simulink model "Projectslxfinal"  (R2021b)
settings: Solver=VariableStepAuto  StartTime=0.0  StopTime=0.01  RelTol=1e-3
undefined symbols (not defined in the file): A_d, B_d, C_d, k, L
libraries: simulink x3, slpidlib x3
settings Model: Creator=hp  LastModifiedBy=mahya
settings DataIOCC: ExternalInput=T1, T2, T3, Gdz1.Numerator{1,1}, Gdz1.Denominator{1,1}, Gdz2.Numerator{1,1}, Gdz2.Denominator{1,1}, Gdz3.Numerator{1,1}, Gdz3.Denominator{1,1}

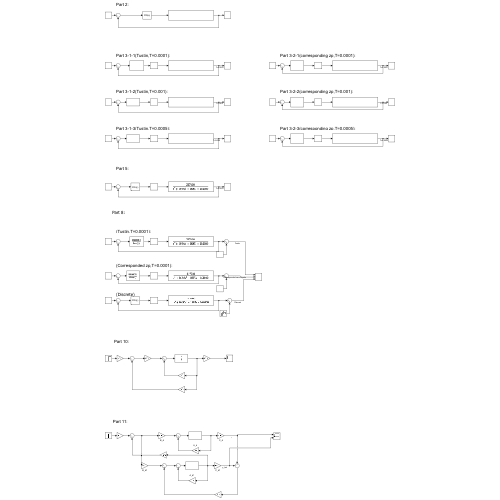
[thumbnail: Simulink's stored preview of the top-level diagram]
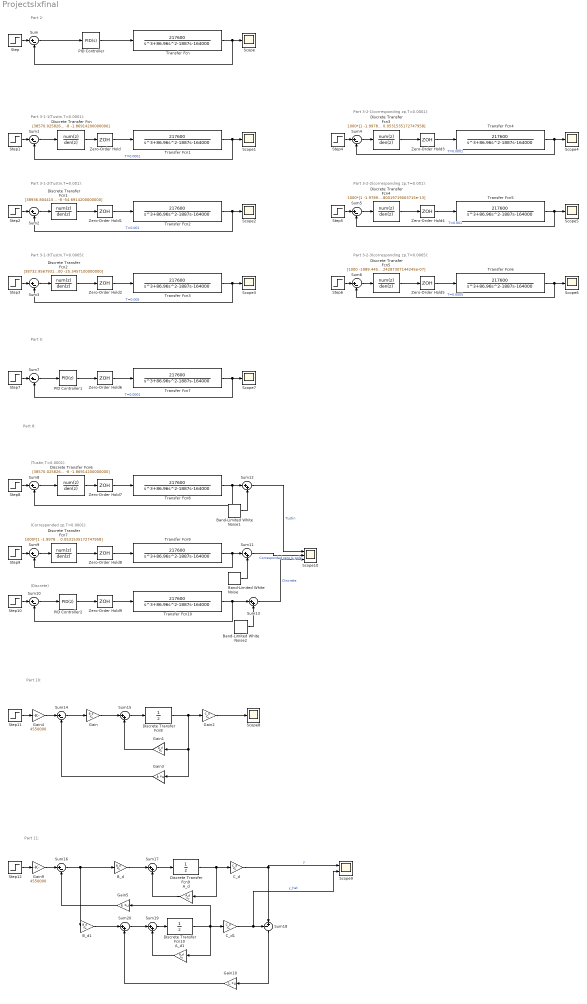
== system Projectslxfinal ==
  note: (Discrete)
  note: Part 8:
  note: Part 5:
  note: Part 2:
  note: Part 3-1-2(Tustin,T=0.001):
  note: Part 3-1-3(Tustin,T=0.0005):
  note: Part 3-2-1(corresponding zp,T=0.0001):
  note: Part 3-1-1(Tustin,T=0.0001):
  note: Part 3-2-2(corresponding zp,T=0.001):
  note: Part 3-2-3(corresponding zp,T=0.0005):
  note: (Corresponded zp,T=0.0001):
  note: (Tustin,T=0.0001):
  note: Part 10:
  note: Part 11:
  A_d : Gain  Gain=A_d  Multiplication=Matrix(K*u)
  A_d1 : Gain  Gain=A_d  Multiplication=Matrix(K*u)
  B_d : Gain  Gain=B_d  Multiplication=Matrix(K*u)
  B_d1 : Gain  Gain=B_d  Multiplication=Matrix(K*u)
  Band-Limited White Noise : simulink/Sources/Band-Limited White Noise  Cov=[0.00001]  Ts=0.1  seed=[23341]
  Band-Limited White Noise1 : simulink/Sources/Band-Limited White Noise  Cov=[0.00001]  Ts=0.1  seed=[23341]
  Band-Limited White Noise2 : simulink/Sources/Band-Limited White Noise  Cov=[0.00001]  Ts=0.1  seed=[23341]
  C_d : Gain  Gain=C_d  Multiplication=Matrix(K*u)
  C_d1 : Gain  Gain=C_d  Multiplication=Matrix(K*u)
  Discrete Transfer Fcn : DiscreteTransferFcn  Numerator=[38570.0258267180 -77058.6188660459 38488.6093872360]  Denominator=[9.86914200000000 -8 -1.86914200000000]  SampleTime=0.0001
  Discrete Transfer Fcn1 : DiscreteTransferFcn  Numerator=[38936.8044151132 -77057.8096445937 38122.6400202932]  Denominator=[62.6914200000000 -8 -54.6914200000000]  SampleTime=0.001
  Discrete Transfer Fcn10 : DiscreteTransferFcn  Denominator=[1 0]
  Discrete Transfer Fcn2 : DiscreteTransferFcn  Numerator=[38732.9567931308 -77058.4226911484 38325.8745957208]  Denominator=[33.3457100000000 -8.00000000000000 -25.3457100000000]  SampleTime=0.0005
  Discrete Transfer Fcn3 : DiscreteTransferFcn  Numerator=1000*[1 -1.99788732081826 0.997889127214699]  Denominator=[1 -1.05315351727480 0.0531535172747958]  SampleTime=0.0001
  Discrete Transfer Fcn4 : DiscreteTransferFcn  Numerator=1000*[1 -1.97891172719588 0.979090657910839]  Denominator=[1 -1.00000000000018 1.80019719003715e-13]  SampleTime=0.001
  Discrete Transfer Fcn5 : DiscreteTransferFcn  Numerator=[1000 -1989.44513045919 989.490099955951]  Denominator=[1 -1.00000042428731 4.24287307144245e-07]  SampleTime=0.0005
  Discrete Transfer Fcn6 : DiscreteTransferFcn  Numerator=[38570.0258267180 -77058.6188660459 38488.6093872360]  Denominator=[9.86914200000000 -8 -1.86914200000000]  SampleTime=0.0001
  Discrete Transfer Fcn7 : DiscreteTransferFcn  Numerator=1000*[1 -1.99788732081826 0.997889127214699]  Denominator=[1 -1.05315351727480 0.0531535172747958]  SampleTime=0.0001
  Discrete Transfer Fcn8 : DiscreteTransferFcn  Denominator=[1 0]
  Discrete Transfer Fcn9 : DiscreteTransferFcn  Denominator=[1 0]
  Gain : Gain  Gain=B_d  Multiplication=Matrix(K*u)
  Gain1 : Gain  Gain=A_d  Multiplication=Matrix(K*u)
  Gain10 : Gain  Gain=L  Multiplication=Matrix(K*u)
  Gain2 : Gain  Gain=C_d  Multiplication=Matrix(K*u)
  Gain3 : Gain  Gain=k  Multiplication=Matrix(K*u)
  Gain4 : Gain  Gain=4550000
  Gain5 : Gain  Gain=k  Multiplication=Matrix(K*u)
  Gain9 : Gain  Gain=4550000
  PID Controller : slpidlib/PID Controller  Controller=PID  Form=Parallel  TimeDomain=Continuous-time  UseExternalTs=off  SampleTime=-1  IntegratorMethod=Forward Euler  FilterMethod=Forward Euler  ControllerParametersSource=internal  P=6.93550294613259  I=13.9271022614454  D=0.32804013853127  UseFilter=on  N=29345.7140521187  TunerSelectOption=Transfer Function Based (PID Tuner App)  ZeroCross=off  InitialConditionSource=internal  InitialConditionForIntegrator=0  InitialConditionForFilter=0  DifferentiatorICPrevScaledInput=0  ExternalReset=none  TrackingMode=off  Kt=1  LimitOutput=off  SatLimitsSource=internal  UpperSaturationLimit=inf  LowerSaturationLimit=-inf  LinearizeAsGain=on  AntiWindupMode=none  Kb=1  POutMin=[]  POutMax=[]  IOutMin=[]  IOutMax=[]  DOutMin=[]  DOutMax=[]  NOutMin=[]  NOutMax=[]  SumOutMin=[]  SumOutMax=[]  SaturationOutMin=[]  SaturationOutMax=[]  PParamMin=[]  PParamMax=[]  IParamMin=[]  IParamMax=[]  DParamMin=[]  DParamMax=[]  NParamMin=[]  NParamMax=[]  KbParamMin=[]  KbParamMax=[]  KtParamMin=[]  KtParamMax=[]  KbOutMin=[]  KbOutMax=[]  KtOutMin=[]  KtOutMax=[]  IntegratorOutMin=[]  IntegratorOutMax=[]  FilterOutMin=[]  FilterOutMax=[]  SumI1OutMin=[]  SumI1OutMax=[]  SumI2OutMin=[]  SumI2OutMax=[]  SumI3OutMin=[]  SumI3OutMax=[]  SumI4OutMin=[]  SumI4OutMax=[]  SumDOutMin=[]  SumDOutMax=[]  DifferentiatorOutMin=[]  DifferentiatorOutMax=[]  FilterDiffOutCoefMin=[]  FilterDiffOutCoefMax=[]  ReciprocalOutMin=[]  ReciprocalOutMax=[]  SumDenOutMin=[]  SumDenOutMax=[]  SumNumOutMin=[]  SumNumOutMax=[]  DivideOutMin=[]  DivideOutMax=[]  UdiffTsProdOutMin=[]  UdiffTsProdOutMax=[]  NTsProdOutMin=[]  NTsProdOutMax=[]  UintegralTsProdOutMin=[]  UintegralTsProdOutMax=[]  UngainTsProdOutMin=[]  UngainTsProdOutMax=[]  IntegratorContinuousStateAttributes=''  IntegratorStateMustResolveToSignalObject=off  IntegratorRTWStateStorageClass=Auto  FilterContinuousStateAttributes=''  FilterStateMustResolveToSignalObject=off  FilterRTWStateStorageClass=Auto  ParallelPVariant=InternalParameters  IdealPVariant=Disabled  IVariant=InternalParameters  DVariant=InternalParameters  IntegratorVariant=Continuous  SatVariant=Disabled  AWVariant=Passthrough  PCopyVariant=Disabled  TRVariant=Disabled  FdbkBlocksVariant=Forward  IdealPFdbkVariant=Disabled  SatFdbkVariant=Disabled  DerivativeFilterVariant=ContFilter  NVariant=InternalParameters  NCopyVariant=Disabled  FilterICVariant=InternalICsFilter  IntegratorICVariant=InternalICs  ExternalResetVariant=Disabled  TRSumVariant=Passthrough  SumFdbkVariant=Disabled  SumVariant=Sum_PID  TsampFilterVariant=InternalTs  TsampNgainVariant=Passthrough  TsampIntegralVariant=Passthrough  ExternalSaturationOutDataTypeStr=Inherit: Same as second input
  PID Controller1 : slpidlib/PID Controller  Controller=PID  Form=Parallel  TimeDomain=Discrete-time  UseExternalTs=off  SampleTime=0.0001  IntegratorMethod=Forward Euler  FilterMethod=Forward Euler  ControllerParametersSource=internal  P=11.3216587748334  I=29.7415043652461  D=0.957335288291549  UseFilter=on  N=14403.0185628453  TunerSelectOption=Transfer Function Based (PID Tuner App)  InitialConditionSource=internal  InitialConditionForIntegrator=0  InitialConditionForFilter=0  DifferentiatorICPrevScaledInput=0  ExternalReset=none  TrackingMode=off  Kt=1  LimitOutput=off  SatLimitsSource=internal  UpperSaturationLimit=inf  LowerSaturationLimit=-inf  LinearizeAsGain=on  AntiWindupMode=none  Kb=1  POutMin=[]  POutMax=[]  IOutMin=[]  IOutMax=[]  DOutMin=[]  DOutMax=[]  NOutMin=[]  NOutMax=[]  SumOutMin=[]  SumOutMax=[]  SaturationOutMin=[]  SaturationOutMax=[]  PParamMin=[]  PParamMax=[]  IParamMin=[]  IParamMax=[]  DParamMin=[]  DParamMax=[]  NParamMin=[]  NParamMax=[]  KbParamMin=[]  KbParamMax=[]  KtParamMin=[]  KtParamMax=[]  KbOutMin=[]  KbOutMax=[]  KtOutMin=[]  KtOutMax=[]  IntegratorOutMin=[]  IntegratorOutMax=[]  FilterOutMin=[]  FilterOutMax=[]  SumI1OutMin=[]  SumI1OutMax=[]  SumI2OutMin=[]  SumI2OutMax=[]  SumI3OutMin=[]  SumI3OutMax=[]  SumI4OutMin=[]  SumI4OutMax=[]  SumDOutMin=[]  SumDOutMax=[]  DifferentiatorOutMin=[]  DifferentiatorOutMax=[]  FilterDiffOutCoefMin=[]  FilterDiffOutCoefMax=[]  ReciprocalOutMin=[]  ReciprocalOutMax=[]  SumDenOutMin=[]  SumDenOutMax=[]  SumNumOutMin=[]  SumNumOutMax=[]  DivideOutMin=[]  DivideOutMax=[]  UdiffTsProdOutMin=[]  UdiffTsProdOutMax=[]  NTsProdOutMin=[]  NTsProdOutMax=[]  UintegralTsProdOutMin=[]  UintegralTsProdOutMax=[]  UngainTsProdOutMin=[]  UngainTsProdOutMax=[]  IntegratorContinuousStateAttributes=''  IntegratorStateMustResolveToSignalObject=off  IntegratorRTWStateStorageClass=Auto  FilterContinuousStateAttributes=''  FilterStateMustResolveToSignalObject=off  FilterRTWStateStorageClass=Auto  ParallelPVariant=InternalParameters  IdealPVariant=Disabled  IVariant=InternalParameters  DVariant=InternalParameters  IntegratorVariant=Discrete  SatVariant=Disabled  AWVariant=Passthrough  PCopyVariant=Disabled  TRVariant=Disabled  FdbkBlocksVariant=Forward  IdealPFdbkVariant=Disabled  SatFdbkVariant=Disabled  DerivativeFilterVariant=ForwardEulerFilter  NVariant=InternalParameters  NCopyVariant=Disabled  FilterICVariant=InternalICsFilter  IntegratorICVariant=InternalICs  ExternalResetVariant=Disabled  TRSumVariant=Passthrough  SumFdbkVariant=Disabled  SumVariant=Sum_PID  TsampFilterVariant=InternalTs  TsampNgainVariant=Passthrough  TsampIntegralVariant=Passthrough  ExternalSaturationOutDataTypeStr=Inherit: Same as second input
  PID Controller2 : slpidlib/PID Controller  Controller=PID  Form=Parallel  TimeDomain=Discrete-time  UseExternalTs=off  SampleTime=0.0001  IntegratorMethod=Forward Euler  FilterMethod=Forward Euler  ControllerParametersSource=internal  P=11.3216587748334  I=29.7415043652461  D=0.957335288291549  UseFilter=on  N=14403.0185628453  TunerSelectOption=Transfer Function Based (PID Tuner App)  InitialConditionSource=internal  InitialConditionForIntegrator=0  InitialConditionForFilter=0  DifferentiatorICPrevScaledInput=0  ExternalReset=none  TrackingMode=off  Kt=1  LimitOutput=off  SatLimitsSource=internal  UpperSaturationLimit=inf  LowerSaturationLimit=-inf  LinearizeAsGain=on  AntiWindupMode=none  Kb=1  POutMin=[]  POutMax=[]  IOutMin=[]  IOutMax=[]  DOutMin=[]  DOutMax=[]  NOutMin=[]  NOutMax=[]  SumOutMin=[]  SumOutMax=[]  SaturationOutMin=[]  SaturationOutMax=[]  PParamMin=[]  PParamMax=[]  IParamMin=[]  IParamMax=[]  DParamMin=[]  DParamMax=[]  NParamMin=[]  NParamMax=[]  KbParamMin=[]  KbParamMax=[]  KtParamMin=[]  KtParamMax=[]  KbOutMin=[]  KbOutMax=[]  KtOutMin=[]  KtOutMax=[]  IntegratorOutMin=[]  IntegratorOutMax=[]  FilterOutMin=[]  FilterOutMax=[]  SumI1OutMin=[]  SumI1OutMax=[]  SumI2OutMin=[]  SumI2OutMax=[]  SumI3OutMin=[]  SumI3OutMax=[]  SumI4OutMin=[]  SumI4OutMax=[]  SumDOutMin=[]  SumDOutMax=[]  DifferentiatorOutMin=[]  DifferentiatorOutMax=[]  FilterDiffOutCoefMin=[]  FilterDiffOutCoefMax=[]  ReciprocalOutMin=[]  ReciprocalOutMax=[]  SumDenOutMin=[]  SumDenOutMax=[]  SumNumOutMin=[]  SumNumOutMax=[]  DivideOutMin=[]  DivideOutMax=[]  UdiffTsProdOutMin=[]  UdiffTsProdOutMax=[]  NTsProdOutMin=[]  NTsProdOutMax=[]  UintegralTsProdOutMin=[]  UintegralTsProdOutMax=[]  UngainTsProdOutMin=[]  UngainTsProdOutMax=[]  IntegratorContinuousStateAttributes=''  IntegratorStateMustResolveToSignalObject=off  IntegratorRTWStateStorageClass=Auto  FilterContinuousStateAttributes=''  FilterStateMustResolveToSignalObject=off  FilterRTWStateStorageClass=Auto  ParallelPVariant=InternalParameters  IdealPVariant=Disabled  IVariant=InternalParameters  DVariant=InternalParameters  IntegratorVariant=Discrete  SatVariant=Disabled  AWVariant=Passthrough  PCopyVariant=Disabled  TRVariant=Disabled  FdbkBlocksVariant=Forward  IdealPFdbkVariant=Disabled  SatFdbkVariant=Disabled  DerivativeFilterVariant=ForwardEulerFilter  NVariant=InternalParameters  NCopyVariant=Disabled  FilterICVariant=InternalICsFilter  IntegratorICVariant=InternalICs  ExternalResetVariant=Disabled  TRSumVariant=Passthrough  SumFdbkVariant=Disabled  SumVariant=Sum_PID  TsampFilterVariant=InternalTs  TsampNgainVariant=Passthrough  TsampIntegralVariant=Passthrough  ExternalSaturationOutDataTypeStr=Inherit: Same as second input
  Scope{,1..8} (9 alike) : Scope
  Scope10 : Scope  NumInputPorts=3
  Scope9 : Scope  NumInputPorts=2
  Step{,1..10,12} (12 alike) : Step  Time=0  SampleTime=0
  Step11 : Step  Time=0  After=2e-3  SampleTime=0
  Sum{,1..10,14,16} (13 alike) : Sum  Inputs=|+-
  Sum{11..13,15,17,19..20} (7 alike) : Sum  Inputs=|++
  Sum18 : Sum  Inputs=-+|
  Transfer Fcn{,1..10} (11 alike) : TransferFcn  Numerator=[217600]  Denominator=[1 86.96 -1887 -164000]
  Zero-Order Hold{,3,6..9} (6 alike) : ZeroOrderHold  SampleTime=0.0001
  Zero-Order Hold1 : ZeroOrderHold  SampleTime=0.001
  Zero-Order Hold2 : ZeroOrderHold  SampleTime=0.0005
  Zero-Order Hold4 : ZeroOrderHold  SampleTime=0.001
  Zero-Order Hold5 : ZeroOrderHold  SampleTime=0.0005
  wires:
  Step/1 -> Sum/1
  Transfer Fcn/1 -> Scope/1, Sum/2
  PID Controller/1 -> Transfer Fcn/1
  Sum/1 -> PID Controller/1
  Sum4/1 -> Discrete Transfer Fcn3/1
  Step4/1 -> Sum4/1
  Zero-Order Hold3/1 -> Transfer Fcn4/1
  Transfer Fcn4/1 -> Scope4/1, Sum4/2  "T=0.0001"
  Zero-Order Hold2/1 -> Transfer Fcn3/1
  Step3/1 -> Sum3/1
  Step2/1 -> Sum2/1
  Transfer Fcn3/1 -> Scope3/1, Sum3/2  "T=0.005"
  Discrete Transfer Fcn1/1 -> Zero-Order Hold1/1
  Zero-Order Hold1/1 -> Transfer Fcn2/1
  Sum3/1 -> Discrete Transfer Fcn2/1
  Sum2/1 -> Discrete Transfer Fcn1/1
  Transfer Fcn2/1 -> Scope2/1, Sum2/2  "T=0.001"
  Transfer Fcn1/1 -> Scope1/1, Sum1/2  "T=0.0001"
  Sum1/1 -> Discrete Transfer Fcn/1
  Step1/1 -> Sum1/1
  Zero-Order Hold/1 -> Transfer Fcn1/1
  Discrete Transfer Fcn/1 -> Zero-Order Hold/1
  Discrete Transfer Fcn2/1 -> Zero-Order Hold2/1
  Discrete Transfer Fcn3/1 -> Zero-Order Hold3/1
  Zero-Order Hold4/1 -> Transfer Fcn5/1
  Step5/1 -> Sum5/1
  Sum5/1 -> Discrete Transfer Fcn4/1
  Discrete Transfer Fcn4/1 -> Zero-Order Hold4/1
  Transfer Fcn5/1 -> Scope5/1, Sum5/2  "T=0.001"
  Zero-Order Hold5/1 -> Transfer Fcn6/1
  Step6/1 -> Sum6/1
  Sum6/1 -> Discrete Transfer Fcn5/1
  Discrete Transfer Fcn5/1 -> Zero-Order Hold5/1
  Transfer Fcn6/1 -> Scope6/1, Sum6/2  "T=0.0005"
  Transfer Fcn7/1 -> Scope7/1, Sum7/2  "T=0.0001"
  Step7/1 -> Sum7/1
  Sum7/1 -> PID Controller1/1
  Zero-Order Hold6/1 -> Transfer Fcn7/1
  PID Controller1/1 -> Zero-Order Hold6/1
  Zero-Order Hold7/1 -> Transfer Fcn8/1
  Sum9/1 -> Discrete Transfer Fcn7/1
  Transfer Fcn9/1 -> Sum11/1, Sum9/2
  Discrete Transfer Fcn6/1 -> Zero-Order Hold7/1
  Discrete Transfer Fcn7/1 -> Zero-Order Hold8/1
  Step9/1 -> Sum9/1
  Transfer Fcn8/1 -> Sum8/2, Sum12/1
  Step8/1 -> Sum8/1
  Zero-Order Hold8/1 -> Transfer Fcn9/1
  Sum8/1 -> Discrete Transfer Fcn6/1
  PID Controller2/1 -> Zero-Order Hold9/1
  Step10/1 -> Sum10/1
  Transfer Fcn10/1 -> Sum13/1, Sum10/2
  Sum10/1 -> PID Controller2/1
  Zero-Order Hold9/1 -> Transfer Fcn10/1
  Band-Limited White Noise/1 -> Sum11/2
  Band-Limited White Noise1/1 -> Sum12/2
  Band-Limited White Noise2/1 -> Sum13/2
  Sum11/1 -> Scope10/2  "Corresponded zero & pole"
  Sum13/1 -> Scope10/3  "Discrete"
  Sum12/1 -> Scope10/1  "Tustin"
  Discrete Transfer Fcn8/1 -> Gain3/1, Gain1/1, Gain2/1
  Gain/1 -> Sum15/1
  Sum15/1 -> Discrete Transfer Fcn8/1
  Gain1/1 -> Sum15/2
  Gain2/1 -> Scope8/1
  Gain3/1 -> Sum14/2
  Sum14/1 -> Gain/1
  Step11/1 -> Gain4/1
  Gain4/1 -> Sum14/1
  Discrete Transfer Fcn9/1 -> A_d/1, C_d/1
  Step12/1 -> Gain9/1
  Sum16/1 -> B_d1/1, B_d/1
  Gain9/1 -> Sum16/1
  Sum17/1 -> Discrete Transfer Fcn9/1
  A_d/1 -> Sum17/2
  C_d/1 -> Sum18/2, Scope9/1  "y"
  B_d/1 -> Sum17/1
  Sum18/1 -> Gain10/1
  Sum19/1 -> Discrete Transfer Fcn10/1
  Discrete Transfer Fcn10/1 -> Gain5/1, A_d1/1, C_d1/1
  A_d1/1 -> Sum19/2
  B_d1/1 -> Sum20/1
  Gain10/1 -> Sum20/2
  Sum20/1 -> Sum19/1
  C_d1/1 -> Scope9/2, Sum18/1  "y_hat"
  Gain5/1 -> Sum16/2
